simulink model "project"  (R2019b)
settings: Solver=VariableStepAuto  StartTime=0.0  StopTime=10.0  RelTol=1e-3
settings Model: Creator=vardhan  LastModifiedBy=vardhan

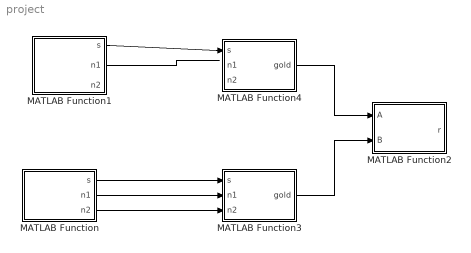
== system project ==
  MATLAB Function : MATLAB Function  TreatAsAtomicUnit=on
  MATLAB Function1 : MATLAB Function  TreatAsAtomicUnit=on
  MATLAB Function2 : MATLAB Function  TreatAsAtomicUnit=on
  MATLAB Function3 : MATLAB Function  TreatAsAtomicUnit=on
  MATLAB Function4 : MATLAB Function  TreatAsAtomicUnit=on
  wires:
  MATLAB Function1/1(s) -> MATLAB Function4/1(s)
  MATLAB Function/1(s) -> MATLAB Function3/1(s)
  MATLAB Function/2(n1) -> MATLAB Function3/2(n1)
  MATLAB Function/3(n2) -> MATLAB Function3/3(n2)
  MATLAB Function4/1(gold) -> MATLAB Function2/1(A)
  MATLAB Function3/1(gold) -> MATLAB Function2/2(B)
  MATLAB Function1/2(n1) -> ?

== matlab function project/MATLAB Function1 ==
  data: s output; n1 output; n2 output
function [s,n1,n2]= fcn
 s=[1 0 1 0 1];
 n1=1;
 n2=3;

== matlab function project/MATLAB Function ==
  data: s output; n1 output; n2 output
function [s,n1,n2]= fcn
 s=[1 0 1 0 1];
 n1=1;
 n2=3;

== matlab function project/MATLAB Function2 ==
  data: A input; r output; B input
function r  = myXCorr(A , B)
N = size(A,2);
M = size(B,2);
r = zeros(1, N + M - 1 );
len = size(r,2);
max_a =max(N,M);
min_a =min(N,M);
for i = 1 : len  
   a = (i - N);
   if(a < 0)
       f = 1;
       l = N + a;
   else
       f = 0;
       l = N - a;
   end
    for j = 1:l
           if(f == 0)
            r(i) = r(i) + A(a + j) * B(j);
           else
            r(i) = r(i) + A(j) * B(j - a);
           end
   end
end
end

== matlab function project/MATLAB Function3 ==
  data: s input; gold output; n1 input; n2 input
function gold = gold_sequence(s,n1,n2)
G=93;  % Code length
x=[];
p1=[];
p2=[];
n=length(s);
%generation of 1st sequence
for j=1:G        
    p1=[p1 s(5)];
    a=xor(s(n1),s(n2));
    s(n-4)=s(n-3);
    s(n-3)=s(n-2);
    s(n-2)=s(n-1);
    s(n-1)=s(n);
    s(n)=a;
end
x=[p1];
%Generation of 2nd sequnces
p2(1)=x(1);
for i=1:30
    j=(3*i)+1;
    p2(i+1)=x(j);
end
%Shifting of p1 in Matrix 'y'
for k=1:31
    for j=1:31
        y(k,j)=x(j+k-1);
    end
end
%Generation of Gold Sequences by modulo 2 sum of p1 and p2
for i=1:31
gold_seq(i,:)=xor(p2,y(i,(1:31)));
end
gold1=reshape(gold_seq,[1,961]);
gold=gold1(1:50);
end

== matlab function project/MATLAB Function4 ==
  data: s input; gold output; n1 input; n2 input
function gold = gold_sequence(s,n1,n2)
G=93;  % Code length
x=[];
p1=[];
p2=[];
n=length(s);
%generation of 1st sequence
for j=1:G        
    p1=[p1 s(5)];
    a=xor(s(n1),s(n2));
    s(n-4)=s(n-3);
    s(n-3)=s(n-2);
    s(n-2)=s(n-1);
    s(n-1)=s(n);
    s(n)=a;
end
x=[p1];
%Generation of 2nd sequnces
p2(1)=x(1);
for i=1:30
    j=(3*i)+1;
    p2(i+1)=x(j);
end
%Shifting of p1 in Matrix 'y'
for k=1:31
    for j=1:31
        y(k,j)=x(j+k-1);
    end
end
%Generation of Gold Sequences by modulo 2 sum of p1 and p2
for i=1:31
gold_seq(i,:)=xor(p2,y(i,(1:31)));
end
gold1=reshape(gold_seq,[1,961]);
gold=gold1(1:50);
end
